simulink model "SAw14_sinusoids_modified"  (Simulink 8.5)
settings: Solver=FixedStepDiscrete  SolverMode=SingleTasking  StartTime=0.0  StopTime=10  RelTol=1e-3
undefined symbols (not defined in the file or in its folder): get
libraries: dspsigops x2, dsparch4 x1, dspspect3 x1, dspsnks4 x1
settings Model: Creator=tanany  LastModifiedBy=DSPadmin
settings DataIOCC: SaveOutput=off  SignalLogging=off  SaveTime=off
settings OptimizationCC: InlineParams=on  ExpressionDepthLimit=128  RollThreshold=2  InitFltsAndDblsToZero=on
settings DebuggingCC: AlgebraicLoopMsg=error  SaveWithParameterizedLinksMsg=none  SignalResolutionControl=TryResolveAllWithWarning  SolverPrmCheckMsg=warning  MultiTaskDSMMsg=warning  MultiTaskCondExecSysMsg=none  SingleTaskRateTransMsg=error  FcnCallInpInsideContextMsg=UseLocalSettings  StateNameClashWarn=none  StrictBusMsg=Warning
settings GRTTargetCC: TargetFcnLib=ansi_tfl_tmw.mat

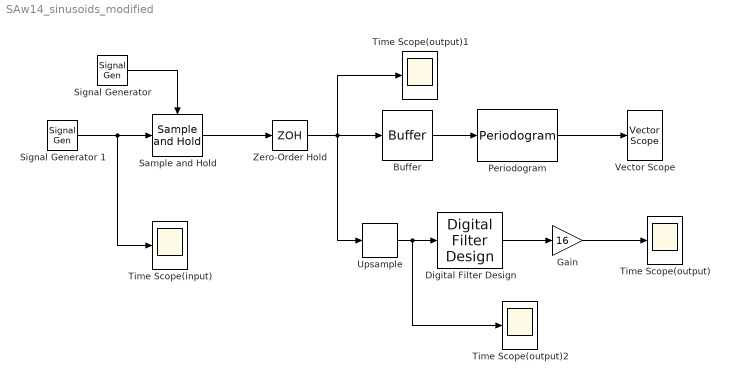
== system SAw14_sinusoids_modified ==
  Buffer : Buffer  N=256
  Digital Filter Design : dsparch4/Digital Filter Design  mwdsp_browser_bugfix_var=off
  Gain : Gain  Gain=16
  Periodogram : dspspect3/Periodogram  measurement=Power spectral density  wintype=Hamming  Rs=50  beta=5  winsamp=Symmetric  FFTImplementation=Auto  inheritFFT=off  fftsize=256  navg=4  inheritTs=on  Ts=1
  Sample and Hold : dspsigops/Sample and Hold  trig=Rising edge  initCond=0  latchinput=off
  "Signal Generator " : SignalGenerator  WaveForm=square  Frequency=1000
  Signal Generator 1 : SignalGenerator  Frequency=100
  Time Scope(input) : Scope
      settings: DataFormat=Structure
  Time Scope(output) : Scope
      settings: DataFormat=Structure
  Time Scope(output)1 : Scope
      settings: SaveName=ScopeData2  DataFormat=Structure
  Time Scope(output)2 : Scope
      settings: SaveName=ScopeData3  DataFormat=Structure
  Upsample : dspsigops/Upsample  N=16  phase=0  InputProcessing=Inherited (this choice will be removed - see release notes)  RateOptions=Allow multirate processing  ic=0  mode=Unused parameter value
  Vector Scope : dspsnks4/Vector Scope  ScopeProperties=on  Domain=Frequency  HorizSpan=1  DisplayProperties=off  AxisGrid=on  Memory=off  FrameNumber=on  AxisLegend=off  AxisZoom=off  OpenScopeAtSimStart=on  OpenScopeImmediately=off  FigPos=get(0,'defaultfigureposition')  AxisProperties=off  XUnits=Hertz  XRange=[0...Fs/2]  InheritXIncr=on  XIncr=1  XLabel=Time  XLimit=Auto  XMin=0  XMax=1  XStart=0  YUnits=dB  YLabel=Amplitude  LineProperties=off  XAxisParamsVer=6.8
      settings: YMin=-47.6422179281401  YMax=16.3758213443065
  Zero-Order Hold : ZeroOrderHold  SampleTime=1/1000
  wires:
  "Signal Generator "/1 -> Sample and Hold/Trigger
  Signal Generator 1/1 -> Sample and Hold/1, Time Scope(input)/1
  Sample and Hold/1 -> Zero-Order Hold/1
  Zero-Order Hold/1 -> Upsample/1, Buffer/1, Time Scope(output)1/1
  Periodogram/1 -> Vector Scope/1
  Upsample/1 -> Digital Filter Design/1, Time Scope(output)2/1
  Digital Filter Design/1 -> Gain/1
  Gain/1 -> Time Scope(output)/1
  Buffer/1 -> Periodogram/1
